simulink model "GNC_integrated"  (R2023a)
settings: Solver=ode4  StartTime=0.0  StopTime=200  FixedStep=0.001  RelTol=1e-3
undefined symbols (not defined in the file or in its folder): Discrete, param, Time
libraries: dspfdesign x20, simulink_extras x6, sharedTrackingLibrary x1, ctrlSharedLib x1, dspmtrx3 x1, SignalEditorBlockLib x1
settings Model: Creator=timme  LastModifiedBy=timme

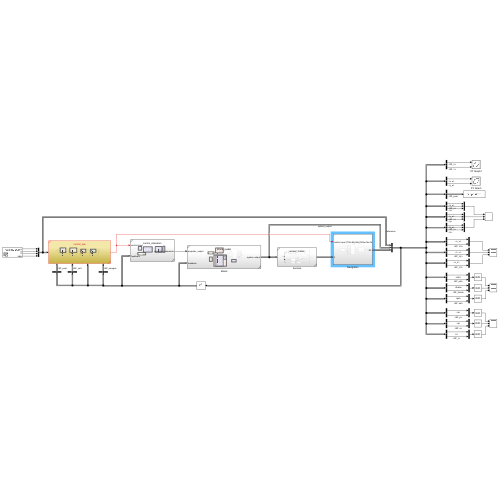
[thumbnail: Simulink's stored preview of the top-level diagram]
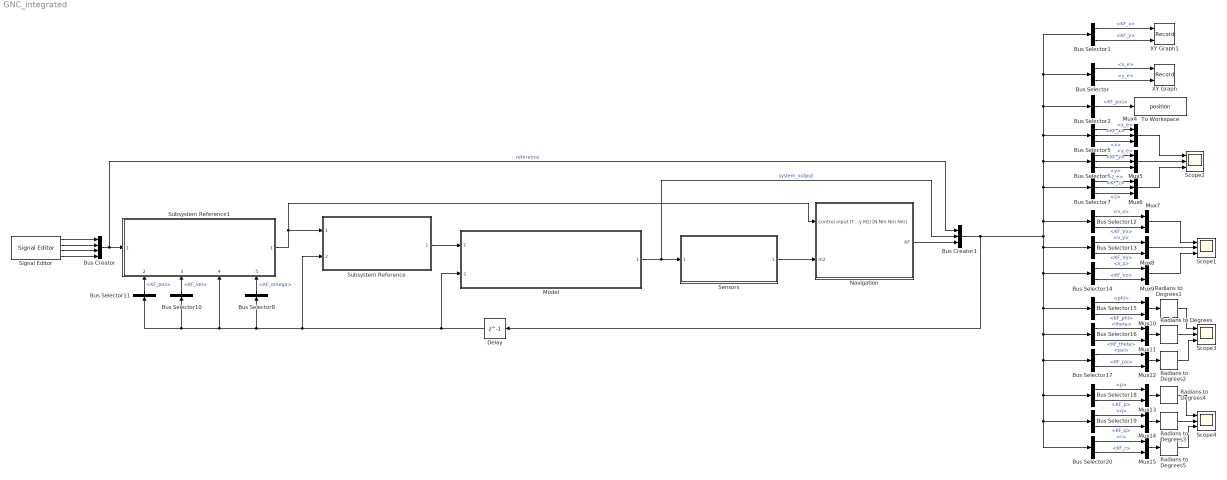
== system GNC_integrated ==
  Bus Creator : BusCreator  Inputs=4
  Bus Creator1 : BusCreator  Inputs=3
  Bus Selector : BusSelector  OutputSignals=system_output.pos.x_e,system_output.pos.y_e
  Bus Selector1 : BusSelector  OutputSignals=x_filt.KF_pos.KF_x,x_filt.KF_pos.KF_y
  Bus Selector10 : BusSelector  OutputSignals=x_filt.KF_vel
  Bus Selector11 : BusSelector  OutputSignals=x_filt.KF_pos
  Bus Selector12 : BusSelector  OutputSignals=system_output.V_e.v_x,x_filt.KF_vel.KF_Vx
  Bus Selector13 : BusSelector  OutputSignals=system_output.V_e.v_y,x_filt.KF_vel.KF_Vy
  Bus Selector14 : BusSelector  OutputSignals=system_output.V_e.v_z,x_filt.KF_vel.KF_Vz
  Bus Selector15 : BusSelector  OutputSignals=system_output.Att.phi,x_filt.KF_att.KF_phi
  Bus Selector16 : BusSelector  OutputSignals=system_output.Att.theta,x_filt.KF_att.KF_theta
  Bus Selector17 : BusSelector  OutputSignals=system_output.Att.psi,x_filt.KF_att.KF_psi
  Bus Selector18 : BusSelector  OutputSignals=system_output.ang_vel.p,x_filt.KF_omega.KF_p
  Bus Selector19 : BusSelector  OutputSignals=system_output.ang_vel.q,x_filt.KF_omega.KF_q
  Bus Selector2 : BusSelector  OutputSignals=x_filt.KF_pos
  Bus Selector20 : BusSelector  OutputSignals=system_output.ang_vel.r,x_filt.KF_omega.KF_r
  Bus Selector5 : BusSelector  OutputSignals=system_output.pos.x_e,x_filt.KF_pos.KF_x,reference.x
  Bus Selector6 : BusSelector  OutputSignals=system_output.pos.y_e,x_filt.KF_pos.KF_y,reference.y
  Bus Selector7 : BusSelector  OutputSignals=system_output.pos.z_e,x_filt.KF_pos.KF_z,reference.z
  Bus Selector8 : BusSelector  OutputSignals=x_filt.KF_omega
  Delay : Delay  DelayLength=1
  Model : Subsystem  ReferencedSubsystem=drone_model
  Mux{7..15} (9 alike) : Mux  Inputs=2
  Mux4 : Mux  Inputs=3
  Mux5 : Mux  Inputs=3
  Mux6 : Mux  Inputs=3
  Navigation : Subsystem
  Radians to Degrees{,1..5} (6 alike) : simulink_extras/Transformations/Radians to Degrees
  Scope{1..4} (4 alike) : Scope  NumInputPorts=3
  Sensors : Subsystem  ReferencedSubsystem=sensor_model
  Signal Editor : SignalEditorBlockLib/Signal Editor  FileName=C:\Users\timme\OneDrive\Bureaublad\Tu Delft\bsc3\DSE\GNC development\Conceptual design phase\Test files\full_system_reference.mat  ActiveScenario=Trajectory_200  ActiveSignal=yaw  IsBus=off  OutputBusObjectStr=Bus: BusObject  SampleTime=param.dt  ZeroCross=off  OutputAfterFinalValue=Setting to zero  Unit=rad  PreserveSignalName=on  ApplySigPropsToAllScenarios=on
  Subsystem Reference : Subsystem  ReferencedSubsystem=control_allocation
  Subsystem Reference1 : Subsystem  ReferencedSubsystem=control_law
      settings: PortSchema="{\"entries\":[{\"content\":{\"sides\":[{\"content\":{\"connectorIds\":[\"In1\"]},\"type\":\"ConnectorPlacement.EquallySpacedRectSide\",\"uuid\":\"cbb659e7-d19a-4e68-9ae7-e5e39426296b\"},{\"content\":{\"connectorIds\":[\"Out1\"],\"side\":\"RIGHT\"},\"type\":\"ConnectorPlacement.EquallySpacedRectSide\",\"uuid\":\"c9f08a4e-80d9-41bf-93e6-4cfd11b32426\"},{\"content\":{\"side\":\"TOP\"},\"type\":\"ConnectorPlacement.EquallySpacedRectSide\",\"uuid\":\"8eafc22d-128e-4ca7-9eba-2c3fd299252c\"},{\"content\":{\"connectorIds\":[\"In2\",\"In3\",\"In4\",\"In5\"],\"side\":\"BOTTOM\"},\"type\":\"ConnectorPlacement.EquallySpacedRectSide\",\"uuid\":\"abe1dc09-e6b8-433e-beaf-ba54ebcb4b47\"}]},\"type\":\"ConnectorPlacement.EquallySpacedConnector\",\"uuid\":\"085ffc95-65e8-4235-be8d-72c324b16b8b\"}],\"packageUris\":[\"http://schema.mathworks.com/mf0/Connector/R2020b\"],\"version\":\"1.0\"}"
  To Workspace : ToWorkspace  VariableName=position  SaveFormat=Timeseries  SampleTime=param.dt
  XY Graph : Record  FileSettingsInternal="{\"entries\":[{\"content\":{\"excelSettings\":{\"content\":{},\"type\":\"Streamout.ExcelSettings\"}},\"type\":\"Streamout.FileSettingStorage\",\"uuid\":\"76f3e39c-791f-414c-bf8e-1f6dbddd9460\"}],\"packageUris\":[\"http://schema.mathworks.com/mf0/streamout_blocks/R2020a\"],\"version\":\"1.0\"}"  Layout=[1 1]  SignalsInternal="{\"entries\":[{\"content\":{},\"type\":\"RecordBlkView.InputSignals\",\"uuid\":\"93fa921d-251e-4d0d-a989-ebcef13dc45f\"}],\"packageUris\":[\"http://schema.mathworks.com/mf0/streamout_blocks/R2020a\"],\"version\":\"1.0\"}"  VisualizationBindings="{\"xyplotplugin\":{\"info\":[{\"series\":[{\"bindingParametersList\":[{\"parameter\":\"X-Axis\",\"signalID\":16,\"signalName\":\"<x_e>\"},{\"parameter\":\"Y-Axis\",\"signalID\":19,\"signalName\":\"<y_e>\"}],\"seriesID\":57418}],\"subplotID\":1}]}}"  CompatibilityTag=XY
  XY Graph1 : Record  FileSettingsInternal="{\"entries\":[{\"content\":{\"excelSettings\":{\"content\":{},\"type\":\"Streamout.ExcelSettings\"}},\"type\":\"Streamout.FileSettingStorage\",\"uuid\":\"e243dce8-001d-48ec-9578-22e94f9af569\"}],\"packageUris\":[\"http://schema.mathworks.com/mf0/streamout_blocks/R2020a\"],\"version\":\"1.0\"}"  Layout=[1 1]  SignalsInternal="{\"entries\":[{\"content\":{},\"type\":\"RecordBlkView.InputSignals\",\"uuid\":\"6a0f3f88-6452-4584-95f5-91d54786c62a\"}],\"packageUris\":[\"http://schema.mathworks.com/mf0/streamout_blocks/R2020a\"],\"version\":\"1.0\"}"  VisualizationBindings="{\"xyplotplugin\":{\"info\":[{\"series\":[{\"bindingParametersList\":[{\"parameter\":\"X-Axis\",\"signalID\":8,\"signalName\":\"<KF_x>\"},{\"parameter\":\"Y-Axis\",\"signalID\":11,\"signalName\":\"<KF_y>\"}],\"seriesID\":58224}],\"subplotID\":1}]}}"  CompatibilityTag=XY
  wires:
  Model/1 -> Sensors/1, Bus Creator1/2  "system_output"
  Bus Selector5/1 -> Mux4/1  "<x_e>"
  Bus Selector5/2 -> Mux4/2  "<KF_x>"
  Bus Selector6/1 -> Mux5/1  "<y_e>"
  Bus Selector6/2 -> Mux5/2  "<KF_y>"
  Bus Selector7/2 -> Mux6/2  "<KF_z>"
  Bus Selector7/1 -> Mux6/1  "<z_e>"
  Bus Selector12/2 -> Mux7/2  "<KF_Vx>"
  Bus Selector12/1 -> Mux7/1  "<v_x>"
  Bus Selector13/1 -> Mux8/1  "<v_y>"
  Bus Selector14/2 -> Mux9/2  "<KF_Vz>"
  Bus Selector14/1 -> Mux9/1  "<v_z>"
  Bus Selector13/2 -> Mux8/2  "<KF_Vy>"
  Bus Selector16/2 -> Mux11/2  "<KF_theta>"
  Mux12/1 -> Radians to Degrees2/1
  Mux11/1 -> Radians to Degrees/1
  Bus Selector17/2 -> Mux12/2  "<KF_psi>"
  Bus Selector17/1 -> Mux12/1  "<psi>"
  Bus Selector15/2 -> Mux10/2  "<KF_phi>"
  Mux10/1 -> Radians to Degrees1/1
  Bus Selector15/1 -> Mux10/1  "<phi>"
  Bus Selector16/1 -> Mux11/1  "<theta>"
  Bus Selector19/2 -> Mux14/2  "<KF_q>"
  Bus Selector18/2 -> Mux13/2  "<KF_p>"
  Mux13/1 -> Radians to Degrees4/1
  Bus Selector20/1 -> Mux15/1  "<r>"
  Bus Selector18/1 -> Mux13/1  "<p>"
  Mux15/1 -> Radians to Degrees5/1
  Bus Selector20/2 -> Mux15/2  "<KF_r>"
  Mux14/1 -> Radians to Degrees3/1
  Bus Selector19/1 -> Mux14/1  "<q>"
  Bus Selector/1 -> XY Graph/1  "<x_e>"
  Bus Selector/2 -> XY Graph/2  "<y_e>"
  Mux5/1 -> Scope2/2
  Mux4/1 -> Scope2/1
  Mux6/1 -> Scope2/3
  Mux8/1 -> Scope1/2
  Mux9/1 -> Scope1/3
  Mux7/1 -> Scope1/1
  Radians to Degrees2/1 -> Scope3/3
  Radians to Degrees1/1 -> Scope3/1
  Radians to Degrees/1 -> Scope3/2
  Radians to Degrees5/1 -> Scope4/3
  Radians to Degrees4/1 -> Scope4/1
  Radians to Degrees3/1 -> Scope4/2
  Bus Selector1/1 -> XY Graph1/1  "<KF_x>"
  Bus Selector1/2 -> XY Graph1/2  "<KF_y>"
  Sensors/1 -> Navigation/2(In2)
  Navigation/1(KF) -> Bus Creator1/3
  Bus Selector2/1 -> To Workspace/1  "<KF_pos>"
  Bus Creator1/1 -> Delay/1, Bus Selector13/1, Bus Selector14/1, Bus Selector20/1, Bus Selector19/1, Bus Selector18/1, Bus Selector17/1, Bus Selector16/1, Bus Selector15/1, Bus Selector12/1, Bus Selector7/1, Bus Selector6/1, Bus Selector2/1, Bus Selector1/1, Bus Selector/1, Bus Selector5/1
  Bus Creator/1 -> Bus Creator1/1, Subsystem Reference1/1  "reference"
  Bus Selector11/1 -> Subsystem Reference1/2  "<KF_pos>"
  Bus Selector10/1 -> Subsystem Reference1/3  "<KF_vel>"
  Delay/1 -> Model/2, Bus Selector8/1, Subsystem Reference1/4, Bus Selector11/1, Bus Selector10/1, Subsystem Reference/2
  Bus Selector8/1 -> Subsystem Reference1/5  "<KF_omega>"
  Subsystem Reference1/1 -> Navigation/1(control input (T Mx My Mz) [N Nm Nm Nm]), Subsystem Reference/1
  Signal Editor/1 -> Bus Creator/1
  Signal Editor/2 -> Bus Creator/2
  Signal Editor/3 -> Bus Creator/3
  Signal Editor/4 -> Bus Creator/4
  Bus Selector5/3 -> Mux4/3  "<x>"
  Bus Selector6/3 -> Mux5/3  "<y>"
  Bus Selector7/3 -> Mux6/3  "<z>"
  Subsystem Reference/1 -> Model/1

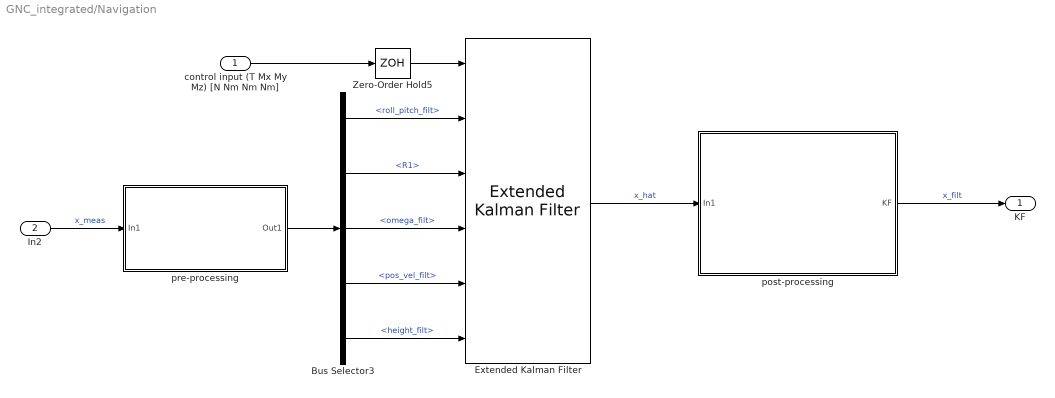
== system GNC_integrated/Navigation ==
  control input (T Mx My Mz) [N Nm Nm Nm] : Inport
  In2 : Inport  Port=2
  Bus Selector3 : BusSelector  OutputSignals=roll_pitch_filt,R1,omega_filt,pos_vel_filt,height_filt
  Extended Kalman Filter : sharedTrackingLibrary/Extended Kalman Filter  StateTransitionFcn=stateTransition  HasStateTransitionJacobianFcn=off  HasAdditiveProcessNoise=Additive  ProcessNoise=diag([1*ones(1,6) [1 1 0.01] [0.1 0.1 0.1]])  HasTimeVaryingProcessNoise=off  HasStateTransitionFcnExtraArgument=1  InitialState=zeros(12,1)  InitialStateCovariance=zeros(12)  MeasurementFcn1=accelerometer_model  HasMeasurementJacobianFcn1=off  HasMeasurementEnablePort1=off  HasAdditiveMeasurementNoise1=Additive  MeasurementNoise1=diag([1 1])  HasTimeVaryingMeasurementNoise1=on  HasMeasurementFcnExtraArgument1=0  HasMeasurementWrapping1=off  MeasurementFcn2=gyrometer_model  HasMeasurementJacobianFcn2=off  HasMeasurementEnablePort2=off  HasAdditiveMeasurementNoise2=Additive  MeasurementNoise2=diag([1 1 10])  HasTimeVaryingMeasurementNoise2=off  HasMeasurementFcnExtraArgument2=0  HasMeasurementWrapping2=off  MeasurementFcn3=GPS_model  HasMeasurementJacobianFcn3=off  HasMeasurementEnablePort3=off  HasAdditiveMeasurementNoise3=Additive  MeasurementNoise3=diag([0.001 0.001 0.001 0.001 0.001 0.001])  HasTimeVaryingMeasurementNoise3=off  HasMeasurementFcnExtraArgument3=0  HasMeasurementWrapping3=off  MeasurementFcn4=Barometer_model  HasMeasurementJacobianFcn4=off  HasMeasurementEnablePort4=off  HasAdditiveMeasurementNoise4=Additive  MeasurementNoise4=0.01  HasTimeVaryingMeasurementNoise4=off  HasMeasurementFcnExtraArgument4=0  HasMeasurementWrapping4=off  MeasurementFcn5=myMeasurementFcn  HasMeasurementJacobianFcn5=off  HasMeasurementEnablePort5=off  HasAdditiveMeasurementNoise5=Additive  MeasurementNoise5=1  HasTimeVaryingMeasurementNoise5=off  HasMeasurementFcnExtraArgument5=0  HasMeasurementWrapping5=off  EnableMultirate=on  StateTransitionFcnSampleTime=0.001  MeasurementFcn1SampleTime=0.001  MeasurementFcn2SampleTime=0.001  MeasurementFcn3SampleTime=0.001  MeasurementFcn4SampleTime=0.01  MeasurementFcn5SampleTime=1  UseCurrentEstimator=on  OutputStateCovariance=off  DataType=double  SampleTime=0.001  NumberOfMeasurements=4
  Zero-Order Hold5 : ZeroOrderHold  SampleTime=0.001
  post-processing : Subsystem
  pre-processing : Subsystem
  KF : Outport
  wires:
  Zero-Order Hold5/1 -> Extended Kalman Filter/1
  In2/1 -> pre-processing/1(In1)  "x_meas"
  control input (T Mx My Mz) [N Nm Nm Nm]/1 -> Zero-Order Hold5/1
  pre-processing/1(Out1) -> Bus Selector3/1
  Bus Selector3/1 -> Extended Kalman Filter/2  "<roll_pitch_filt>"
  Bus Selector3/3 -> Extended Kalman Filter/4  "<omega_filt>"
  Bus Selector3/4 -> Extended Kalman Filter/5  "<pos_vel_filt>"
  Bus Selector3/5 -> Extended Kalman Filter/6  "<height_filt>"
  Bus Selector3/2 -> Extended Kalman Filter/3  "<R1>"
  Extended Kalman Filter/1 -> post-processing/1(In1)  "x_hat"
  post-processing/1(KF) -> KF/1  "x_filt"

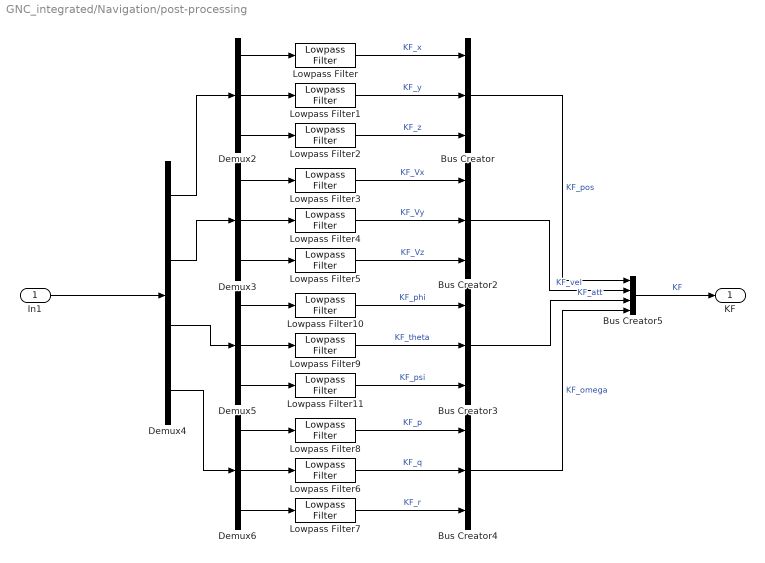
== system GNC_integrated/Navigation/post-processing ==
  In1 : Inport
  Bus Creator{,2..4} (4 alike) : BusCreator  Inputs=3
  Bus Creator5 : BusCreator  Inputs=4
  Demux{2..3,5..6} (4 alike) : Demux  Outputs=3
  Demux4 : Demux
  Lowpass Filter{,1..5,9..11} (9 alike) : dspfdesign/Lowpass Filter  FilterType=IIR  DesignForMinimumOrder=on  FilterOrder=50  PassbandFrequency=1  StopbandFrequency=499  PassbandRipple=0.1  StopbandAttenuation=50  SampleRateMode=Specify on dialog  SampleRate=1000  SimulateUsing=Interpreted execution  roundingMode=Floor  coeffsDataTypeStr=fixdt(1,16)
  Lowpass Filter6 : dspfdesign/Lowpass Filter  FilterType=IIR  DesignForMinimumOrder=on  FilterOrder=50  PassbandFrequency=5  StopbandFrequency=100  PassbandRipple=0.1  StopbandAttenuation=45  SampleRateMode=Specify on dialog  SampleRate=1000  SimulateUsing=Interpreted execution  roundingMode=Floor  coeffsDataTypeStr=fixdt(1,16)
  Lowpass Filter7 : dspfdesign/Lowpass Filter  FilterType=IIR  DesignForMinimumOrder=on  FilterOrder=50  PassbandFrequency=5  StopbandFrequency=100  PassbandRipple=0.1  StopbandAttenuation=45  SampleRateMode=Specify on dialog  SampleRate=1000  SimulateUsing=Interpreted execution  roundingMode=Floor  coeffsDataTypeStr=fixdt(1,16)
  Lowpass Filter8 : dspfdesign/Lowpass Filter  FilterType=IIR  DesignForMinimumOrder=on  FilterOrder=50  PassbandFrequency=5  StopbandFrequency=100  PassbandRipple=0.1  StopbandAttenuation=45  SampleRateMode=Specify on dialog  SampleRate=1000  SimulateUsing=Interpreted execution  roundingMode=Floor  coeffsDataTypeStr=fixdt(1,16)
  KF : Outport
  wires:
  Demux3/1 -> Lowpass Filter3/1
  Lowpass Filter/1 -> Bus Creator/1  "KF_x"
  Lowpass Filter1/1 -> Bus Creator/2  "KF_y"
  Demux2/2 -> Lowpass Filter1/1
  Demux2/1 -> Lowpass Filter/1
  Demux4/4 -> Demux6/1
  Demux2/3 -> Lowpass Filter2/1
  Lowpass Filter3/1 -> Bus Creator2/1  "KF_Vx"
  Bus Creator/1 -> Bus Creator5/1  "KF_pos"
  Lowpass Filter5/1 -> Bus Creator2/3  "KF_Vz"
  Bus Creator3/1 -> Bus Creator5/3  "KF_att"
  Lowpass Filter9/1 -> Bus Creator3/2  "KF_theta"
  Demux3/3 -> Lowpass Filter5/1
  Demux4/2 -> Demux3/1
  Lowpass Filter6/1 -> Bus Creator4/2  "KF_q"
  Demux3/2 -> Lowpass Filter4/1
  Demux4/3 -> Demux5/1
  Demux4/1 -> Demux2/1
  Lowpass Filter2/1 -> Bus Creator/3  "KF_z"
  Bus Creator4/1 -> Bus Creator5/4  "KF_omega"
  Lowpass Filter10/1 -> Bus Creator3/1  "KF_phi"
  Demux6/2 -> Lowpass Filter6/1
  Lowpass Filter7/1 -> Bus Creator4/3  "KF_r"
  Demux5/1 -> Lowpass Filter10/1
  Bus Creator2/1 -> Bus Creator5/2  "KF_vel"
  Demux5/2 -> Lowpass Filter9/1
  Demux6/1 -> Lowpass Filter8/1
  Lowpass Filter8/1 -> Bus Creator4/1  "KF_p"
  Demux6/3 -> Lowpass Filter7/1
  Lowpass Filter4/1 -> Bus Creator2/2  "KF_Vy"
  Bus Creator5/1 -> KF/1  "KF"
  Demux5/3 -> Lowpass Filter11/1
  Lowpass Filter11/1 -> Bus Creator3/3  "KF_psi"
  In1/1 -> Demux4/1

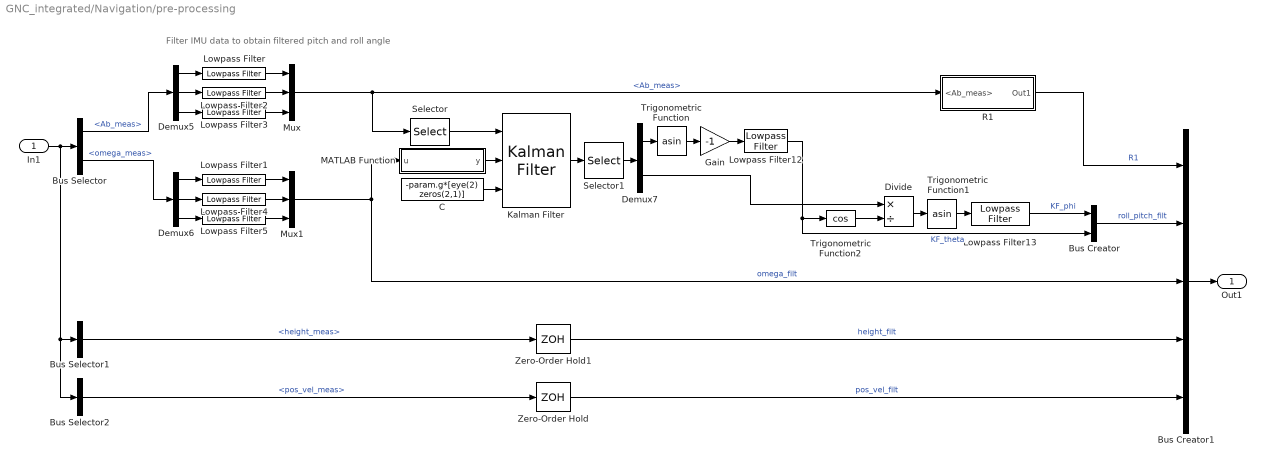
== system GNC_integrated/Navigation/pre-processing ==
  note: Filter IMU data to obtain filtered pitch and roll angle
  In1 : Inport
  Bus Creator : BusCreator  Inputs=2
  Bus Creator1 : BusCreator  Inputs=5
  Bus Selector : BusSelector  OutputSignals=Ab_meas,omega_meas
  Bus Selector1 : BusSelector  OutputSignals=height_meas
  Bus Selector2 : BusSelector  OutputSignals=pos_vel_meas
  C : Constant  Value=-param.g*[eye(2) zeros(2,1)]  SampleTime=0.001
  Demux5 : Demux  Outputs=3
  Demux6 : Demux  Outputs=3
  Demux7 : Demux  Outputs=2
  Divide : Product  Inputs=*/
  Gain : Gain  Gain=-1
  Kalman Filter : ctrlSharedLib/Kalman Filter  TimeDomain=Discrete-Time  UseCurrentEstimator=on  ModelSource=Input port  ModelSourceVariable=ss(0.95,1,1,0,1)  A=0.95  B=1  C=1  D=0  NumberOfStates=3  NumberOfInputs=1  NumberOfOutputs=2  InitialEstimateSource=Dialog  X0=0  P0=1  UseK=off  UseGH=off  NumberOfProcessNoiseInputs=1  G=eye(3)  TimeInvariantG=on  H=ones(2,1)  TimeInvariantH=on  Q=100  TimeInvariantQ=on  R=0.0001  TimeInvariantR=on  N=0  TimeInvariantN=on  AddInputPort=off  AddEnablePort=off  OutputEstimatedY=off  OutputP=off  Ts=0.001
  Lowpass Filter : dspfdesign/Lowpass Filter  FilterType=IIR  DesignForMinimumOrder=on  FilterOrder=50  PassbandFrequency=50  StopbandFrequency=499  PassbandRipple=0.1  StopbandAttenuation=80  SampleRateMode=Specify on dialog  SampleRate=1000  SimulateUsing=Interpreted execution  roundingMode=Floor  coeffsDataTypeStr=fixdt(1,16)
  Lowpass Filter1 : dspfdesign/Lowpass Filter  FilterType=IIR  DesignForMinimumOrder=on  FilterOrder=50  PassbandFrequency=25  StopbandFrequency=499  PassbandRipple=0.1  StopbandAttenuation=80  SampleRateMode=Specify on dialog  SampleRate=1000  SimulateUsing=Interpreted execution  roundingMode=Floor  coeffsDataTypeStr=fixdt(1,16)
  Lowpass Filter12 : dspfdesign/Lowpass Filter  FilterType=IIR  DesignForMinimumOrder=on  FilterOrder=50  PassbandFrequency=5  StopbandFrequency=60  PassbandRipple=0.1  StopbandAttenuation=45  SampleRateMode=Specify on dialog  SampleRate=1000  SimulateUsing=Interpreted execution  roundingMode=Floor  coeffsDataTypeStr=fixdt(1,16)
  Lowpass Filter13 : dspfdesign/Lowpass Filter  FilterType=IIR  DesignForMinimumOrder=on  FilterOrder=50  PassbandFrequency=5  StopbandFrequency=60  PassbandRipple=0.1  StopbandAttenuation=45  SampleRateMode=Specify on dialog  SampleRate=1000  SimulateUsing=Interpreted execution  roundingMode=Floor  coeffsDataTypeStr=fixdt(1,16)
  Lowpass Filter2 : dspfdesign/Lowpass Filter  FilterType=IIR  DesignForMinimumOrder=on  FilterOrder=50  PassbandFrequency=50  StopbandFrequency=499  PassbandRipple=0.1  StopbandAttenuation=80  SampleRateMode=Specify on dialog  SampleRate=1000  SimulateUsing=Interpreted execution  roundingMode=Floor  coeffsDataTypeStr=fixdt(1,16)
  Lowpass Filter3 : dspfdesign/Lowpass Filter  FilterType=IIR  DesignForMinimumOrder=on  FilterOrder=50  PassbandFrequency=50  StopbandFrequency=499  PassbandRipple=0.1  StopbandAttenuation=80  SampleRateMode=Specify on dialog  SampleRate=1000  SimulateUsing=Interpreted execution  roundingMode=Floor  coeffsDataTypeStr=fixdt(1,16)
  Lowpass Filter4 : dspfdesign/Lowpass Filter  FilterType=IIR  DesignForMinimumOrder=on  FilterOrder=50  PassbandFrequency=25  StopbandFrequency=499  PassbandRipple=0.1  StopbandAttenuation=80  SampleRateMode=Specify on dialog  SampleRate=1000  SimulateUsing=Interpreted execution  roundingMode=Floor  coeffsDataTypeStr=fixdt(1,16)
  Lowpass Filter5 : dspfdesign/Lowpass Filter  FilterType=IIR  DesignForMinimumOrder=on  FilterOrder=50  PassbandFrequency=25  StopbandFrequency=499  PassbandRipple=0.1  StopbandAttenuation=80  SampleRateMode=Specify on dialog  SampleRate=1000  SimulateUsing=Interpreted execution  roundingMode=Floor  coeffsDataTypeStr=fixdt(1,16)
  MATLAB Function : MATLAB Function  TreatAsAtomicUnit=on
  Mux : Mux  Inputs=3
  Mux1 : Mux  Inputs=3
  R1 : Subsystem
  Selector : Selector  InputPortWidth=3  IndexOptions=Index vector (dialog)  Indices=[1 2]  OutputSizes=1
  Selector1 : Selector  InputPortWidth=3  IndexOptions=Index vector (dialog)  Indices=[1 2]  OutputSizes=1
  Trigonometric Function : Trigonometry  Operator=asin
  Trigonometric Function1 : Trigonometry  Operator=asin
  Trigonometric Function2 : Trigonometry  Operator=cos
  Zero-Order Hold : ZeroOrderHold  SampleTime=0.001
  Zero-Order Hold1 : ZeroOrderHold  SampleTime=0.01
  Out1 : Outport
  wires:
  MATLAB Function/1(y) -> Kalman Filter/2
  Divide/1 -> Trigonometric Function1/1
  Trigonometric Function1/1 -> Lowpass Filter13/1
  Trigonometric Function2/1 -> Divide/2
  Bus Selector/2 -> Demux6/1  "<omega_meas>"
  Bus Selector/1 -> Demux5/1  "<Ab_meas>"
  Lowpass Filter12/1 -> Trigonometric Function2/1, Bus Creator/2  "KF_theta"
  Selector/1 -> Kalman Filter/1
  Demux7/1 -> Trigonometric Function/1
  Gain/1 -> Lowpass Filter12/1
  C/1 -> Kalman Filter/3
  Trigonometric Function/1 -> Gain/1
  Kalman Filter/1 -> Selector1/1
  Selector1/1 -> Demux7/1
  Demux7/2 -> Divide/1
  Lowpass Filter13/1 -> Bus Creator/1  "KF_phi"
  In1/1 -> Bus Selector2/1, Bus Selector1/1, Bus Selector/1
  Demux6/1 -> Lowpass Filter1/1
  Lowpass Filter3/1 -> Mux/3
  Lowpass Filter4/1 -> Mux1/2
  Lowpass Filter1/1 -> Mux1/1
  Demux5/3 -> Lowpass Filter3/1
  Lowpass Filter2/1 -> Mux/2
  Demux6/3 -> Lowpass Filter5/1
  Demux5/2 -> Lowpass Filter2/1
  Lowpass Filter5/1 -> Mux1/3
  Lowpass Filter/1 -> Mux/1
  Demux6/2 -> Lowpass Filter4/1
  Demux5/1 -> Lowpass Filter/1
  Mux1/1 -> Bus Creator1/3, MATLAB Function/1(u)  "omega_filt"
  Bus Creator1/1 -> Out1/1
  Bus Selector1/1 -> Zero-Order Hold1/1  "<height_meas>"
  Bus Creator/1 -> Bus Creator1/2  "roll_pitch_filt"
  Bus Selector2/1 -> Zero-Order Hold/1  "<pos_vel_meas>"
  Zero-Order Hold/1 -> Bus Creator1/5  "pos_vel_filt"
  Zero-Order Hold1/1 -> Bus Creator1/4  "height_filt"
  Mux/1 -> R1/1(<Ab_meas>), Selector/1  "<Ab_meas>"
  R1/1(Out1) -> Bus Creator1/1  "R1"

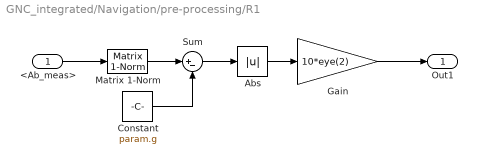
== system GNC_integrated/Navigation/pre-processing/R1 ==
  <Ab_meas> : Inport
  Abs : Abs  SaturateOnIntegerOverflow=off
  Constant : Constant  Value=param.g
  Gain : Gain  Gain=10*eye(2)
  Matrix 1-Norm : dspmtrx3/Matrix  1-Norm  roundingMode=Floor  overflowMode=off  outputDataTypeStr=Inherit: Same as accumulator  outputMin=[]  outputMax=[]  outputLastDataTypeStr=Inherit: Same as accumulator
  Sum : Sum  Inputs=|+-
  Out1 : Outport
  wires:
  Matrix 1-Norm/1 -> Sum/1
  <Ab_meas>/1 -> Matrix 1-Norm/1
  Constant/1 -> Sum/2
  Sum/1 -> Abs/1
  Gain/1 -> Out1/1
  Abs/1 -> Gain/1

== matlab function GNC_integrated/Navigation/pre-processing/MATLAB Function ==
  data: u input; y output
function y = fcn(u)

y = -[0 -u(3) u(2) ; u(3) 0 -u(1) ; -u(2) u(1) 0 ];
